simulink model "mass_spring_damper"  (R2022b)
settings: Solver=VariableStepAuto  StartTime=0.0  StopTime=10.0  RelTol=1e-3
settings Model: Creator=Moham  LastModifiedBy=Moham

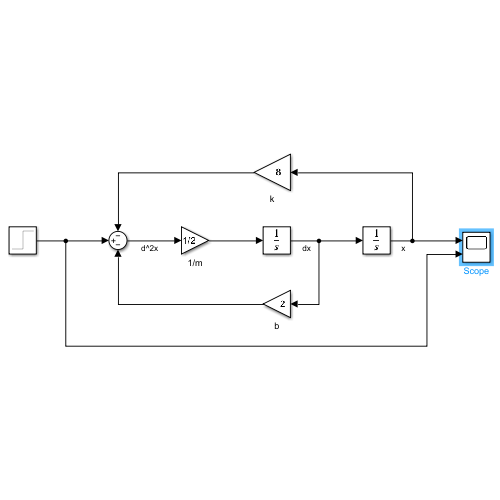
[thumbnail: Simulink's stored preview of the top-level diagram]
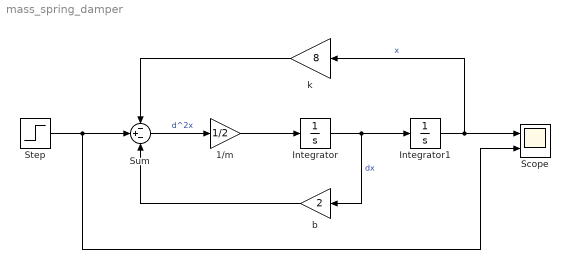
== system mass_spring_damper ==
  1/m : Gain  Gain=1/2
  Integrator : Integrator
  Integrator1 : Integrator
  Scope : Scope  NumInputPorts=2
  Step : Step  SampleTime=0
  Sum : Sum  Inputs=-+-
  b : Gain  Gain=2
  k : Gain  Gain=8
  wires:
  Integrator/1 -> b/1, Integrator1/1  "dx"
  1/m/1 -> Integrator/1
  Integrator1/1 -> k/1, Scope/1  "x"
  Sum/1 -> 1/m/1  "d^2x"
  Step/1 -> Scope/2, Sum/2
  k/1 -> Sum/1
  b/1 -> Sum/3
